simulink model "untitledyeni"  (R2023b)
settings: Solver=VariableStepAuto  StartTime=0.0  StopTime=1  RelTol=1e-3
libraries: dspsigops x1, dspquant2 x1
settings Model: Creator=Mustafa  LastModifiedBy=Mustafa

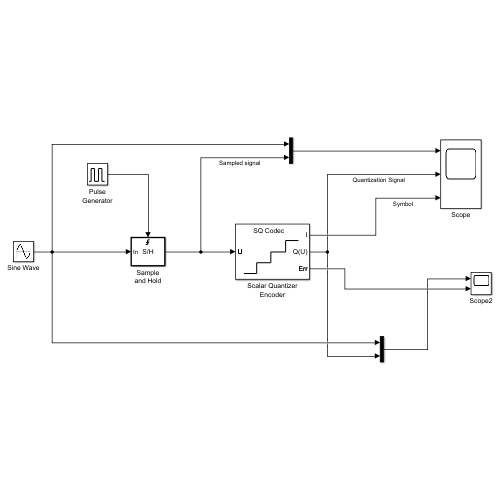
[thumbnail: Simulink's stored preview of the top-level diagram]
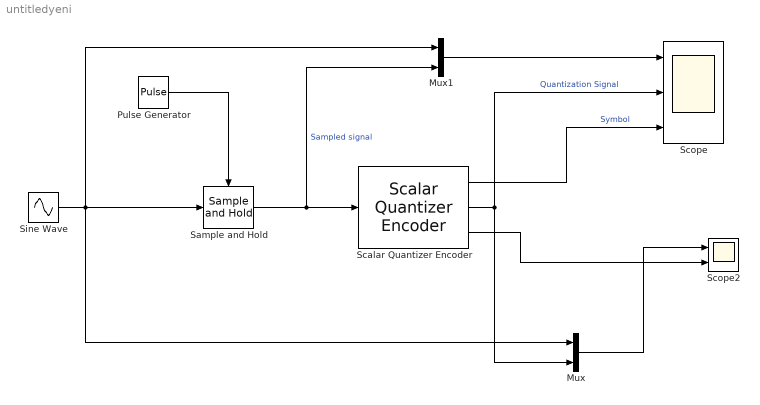
== system untitledyeni ==
  Mux : Mux  Inputs=2
  Mux1 : Mux  Inputs=2
  Pulse Generator : DiscretePulseGenerator  PulseType=Time based  Period=1/10  PulseWidth=5
  Sample and Hold : dspsigops/Sample and Hold  trig=Rising edge  initCond=0  latchinput=off
  Scalar Quantizer Encoder : dspquant2/Scalar Quantizer Encoder  paramSrc=Specify via dialog  partType=Bounded  BBoundary=[-1 -0.5 0 0.5 1]  UBoundary=[2:9]  SearchMethod=Linear  tieBreakRule=Choose the lower index  outQU=on  outQError=on  codebook=[-0.75 -0.25 0.25 0.75]  outStatus=off  invalidin=Clip  idtype=Inherit via back propagation  roundingMode=Floor  overflowMode=off
  Scope : Scope  NumInputPorts=3
  Scope2 : Scope  NumInputPorts=2
  Sine Wave : Sin  Frequency=2*pi*1  Phase=pi/2  SampleTime=0
  wires:
  Mux/1 -> Scope2/1
  Sine Wave/1 -> Mux1/1, Mux/1, Sample and Hold/1
  Sample and Hold/1 -> Scalar Quantizer Encoder/1, Mux1/2  "Sampled signal"
  Mux1/1 -> Scope/1
  Scalar Quantizer Encoder/3 -> Scope2/2
  Scalar Quantizer Encoder/2 -> Scope/2, Mux/2  "Quantization Signal"
  Scalar Quantizer Encoder/1 -> Scope/3  "Symbol"
  Pulse Generator/1 -> Sample and Hold/Trigger
